simulink model "VOO"  (R2022a)
settings: Solver=FixedStepAuto  StartTime=0.0  StopTime=10.0  FixedStep=1e-3  RelTol=1e-3  EnableMultiTasking=on
undefined symbols (not defined in the file): D10, D11, D12, D2, D4, D5, D7, D8, D9, PTA0, PTA2, PTB23, PTB9, PTC3, PTC4, PTD0, PTD2, PTD3
libraries: frdmk64flib x10
settings Model: ExtModeTrigDuration=5  Creator=jacqu  LastModifiedBy=jacqu
settings OptimizationCC: EnhancedBackFolding=on  PassReuseOutputArgsAs=Individual arguments  ZeroExternalMemoryAtStartup=off  ZeroInternalMemoryAtStartup=off  MaxStackSize=64  OptimizeBlockOrder=speed  DifferentSizesBufferReuse=on  OptimizationCustomize=off  EfficientTunableParamExpr=on
settings DebuggingCC: ParameterTunabilityLossMsg=error
settings HardwareCC: ProdBitPerPointer=32  ProdBitPerSizeT=32  ProdBitPerPtrDiffT=32  ProdLargestAtomicInteger=Long  ProdLargestAtomicFloat=Double  ProdWordSize=32  ProdHWDeviceType=ARM Compatible->ARM Cortex
settings SFSimCC: MATLABDynamicMemAlloc=off
settings RTWCC: SystemTargetFile=ert.tlc  HardwareBoard=NXP FRDM-K64F  TLCOptions="-aInlineSetEventsForThisBaseRateFcn=TLC_FALSE -aSuppressMultiTaskScheduler=TLC_FALSE  -aRateBasedStepFcn=0"  TemplateMakefile=ert_default_tmf  Toolchain=GNU Tools for ARM Embedded Processors
settings CodeAppCC: ForceParamTrailComments=on  IgnoreCustomStorageClasses=off  OperatorAnnotations=on  SimulinkDataObjDesc=on  SFDataObjDesc=on  InsertBlockDesc=on
settings ERTTargetCC: ExtModeTransport=4  ExtModeMexFile=sendToCommService

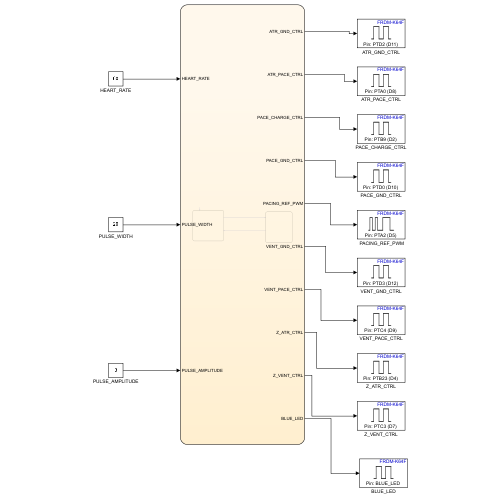
[thumbnail: Simulink's stored preview of the top-level diagram]
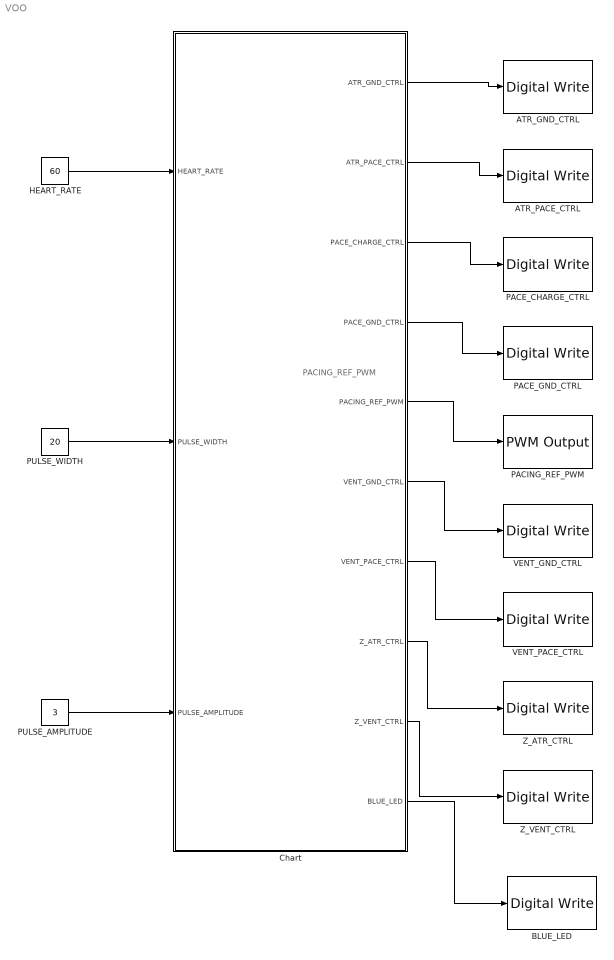
== system VOO ==
  note: PACING_REF_PWM
  " PACING_REF_PWM" : frdmk64flib/PWM Output  Whichpin=PTA2 (D5)  InitialFrequency=2000  InitialDutyCycle=50
  ATR_GND_CTRL : frdmk64flib/Digital Write  Whichpin=PTD2 (D11)
  ATR_PACE_CTRL : frdmk64flib/Digital Write  Whichpin=PTA0 (D8)
  BLUE_LED : frdmk64flib/Digital Write  Whichpin=BLUE_LED
  Chart : Stateflow chart  TreatAsAtomicUnit=on
  HEART_RATE : Constant  Value=60
  PACE_CHARGE_CTRL : frdmk64flib/Digital Write  Whichpin=PTB9 (D2)
  PACE_GND_CTRL : frdmk64flib/Digital Write  Whichpin=PTD0 (D10)
  PULSE_AMPLITUDE : Constant  Value=3
  PULSE_WIDTH : Constant  Value=20
  VENT_GND_CTRL : frdmk64flib/Digital Write  Whichpin=PTD3 (D12)
  VENT_PACE_CTRL : frdmk64flib/Digital Write  Whichpin=PTC4 (D9)
  Z_ATR_CTRL : frdmk64flib/Digital Write  Whichpin=PTB23 (D4)
  Z_VENT_CTRL : frdmk64flib/Digital Write  Whichpin=PTC3 (D7)
  wires:
  Chart/1(ATR_GND_CTRL) -> ATR_GND_CTRL/1
  Chart/6(VENT_GND_CTRL) -> VENT_GND_CTRL/1
  Chart/2(ATR_PACE_CTRL) -> ATR_PACE_CTRL/1
  Chart/4(PACE_GND_CTRL) -> PACE_GND_CTRL/1
  Chart/8(Z_ATR_CTRL) -> Z_ATR_CTRL/1
  HEART_RATE/1 -> Chart/1(HEART_RATE)
  PULSE_WIDTH/1 -> Chart/2(PULSE_WIDTH)
  Chart/5(PACING_REF_PWM) -> " PACING_REF_PWM"/1
  Chart/3(PACE_CHARGE_CTRL) -> PACE_CHARGE_CTRL/1
  Chart/7(VENT_PACE_CTRL) -> VENT_PACE_CTRL/1
  PULSE_AMPLITUDE/1 -> Chart/3(PULSE_AMPLITUDE)
  Chart/9(Z_VENT_CTRL) -> Z_VENT_CTRL/1
  Chart/10(BLUE_LED) -> BLUE_LED/1

== stateflow chart VOO/Chart ==
  state PACE_OFF
    entry:
    ATR_PACE_CTRL = 0
    VENT_PACE_CTRL = 0
    PACING_REF_PWM = 20*PULSE_AMPLITUDE
    PACE_CHARGE_CTRL = 1
    PACE_GND_CTRL = 1
    VENT_PACE_CTRL = 0
    Z_ATR_CTRL = 0
    Z_VENT_CTRL = 0
    ATR_PACE_CTRL = 0
    ATR_GND_CTRL = 0
    VENT_GND_CTRL = 1
    BLUE_LED = 0
  state PACE_ON
    entry:
    PACE_CHARGE_CTRL = 0
    PACE_GND_CTRL = 1
    ATR_PACE_CTRL = 0
    ATR_GND_CTRL = 0
    Z_ATR_CTRL = 0
    Z_VENT_CTRL = 0
    VENT_GND_CTRL = 0
    VENT_PACE_CTRL = 1
    BLUE_LED = 1
  (default) -> PACE_OFF
  PACE_OFF -> PACE_ON : [after((60000/HEART_RATE)-PULSE_WIDTH,msec)]
  PACE_ON -> PACE_OFF : [after(PULSE_WIDTH,msec)]
  data: HEART_RATE input; PULSE_WIDTH input; PULSE_AMPLITUDE input; ATR_GND_CTRL output; ATR_PACE_CTRL output; PACE_CHARGE_CTRL output; PACE_GND_CTRL output; PACING_REF_PWM output; VENT_GND_CTRL output; VENT_PACE_CTRL output; Z_ATR_CTRL output; Z_VENT_CTRL output; BLUE_LED output
